simulink model "psbfilter"  (Simulink 6.0)
settings: Solver=ode45  SolverMode=SingleTasking  StartTime=0.0  StopTime=0.1  RelTol=1e-3  AbsTol=1e-6
libraries: powerlib2 x14
settings Model: Creator=patrice  LastModifiedBy=batserve  ExtModeTrigMode=oneshot  ExtModeArmWhenConnect=off  ExtModeAutoUpdateStatusClock=off
settings DataIOCC: LimitDataPoints=off  SignalLoggingName=sigsOut
settings OptimizationCC: BlockReduction=off  BooleanDataType=off
settings DebuggingCC: CheckExecutionContextPreStartOutputMsg=on  CheckExecutionContextRuntimeOutputMsg=on  SolverPrmCheckMsg=none
settings HardwareCC: TargetUnknown=on
settings RTWCC: TemplateMakefile=grt_unix.tmf

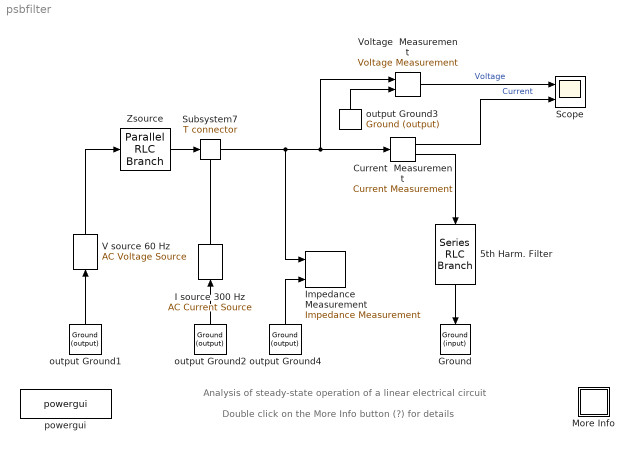
== system psbfilter ==
  note: Analysis of steady-state operation of a linear electrical circuit
  note: Double click on the More Info button (?) for details
  5th Harm. Filter : powerlib2/Elements/Series RLC Branch  Tag=PoWeRsYsTeMbLoCk  Orientation=down  a=1.27  b=107.42e-03  c=2.62e-06  mesure=None  PSBOutputType=1
  Current  Measurement : powerlib2/Measurements/Current Measurement  Tag=PoWeRsYsTeMmEaSuReMeNt  PhasorSimulation=off  OutputType=Magnitude  PSBOutputType=01  PSBequivalent=0
  Ground : powerlib2/Connectors/Ground (input)  Tag=PoWeRsYsTeMbLoCk  Orientation=down
  I source 300 Hz : powerlib2/Electrical Sources/AC Current Source  Tag=PoWeRsYsTeMbLoCk  Orientation=up  A=10  P=-30  F=300  stime=0  mesure=None  PSBOutputType=1
  Impedance  Measurement : powerlib2/Measurements/Impedance Measurement  Tag=PoWeRsYsTeMbLoCk  kz=1
  More Info : Subsystem
      mask Display: disp('?')
  Scope : Scope  NumInputPorts=2
      settings: TimeRange=0.1  YMin=-200~-10  YMax=200~10  DataFormat=Array
  Subsystem7 : powerlib2/Connectors/T connector  Tag=PoWeRsYsTeMbLoCk  PSBOutputType=1
  V source 60 Hz : powerlib2/Electrical Sources/AC Voltage Source  Tag=PoWeRsYsTeMbLoCk  Orientation=up  A=100  P=0  F=60  stime=0  mesure=None  PSBOutputType=1
  Voltage  Measurement : powerlib2/Measurements/Voltage Measurement  Tag=PoWeRsYsTeMmEaSuReMeNt  PhasorSimulation=off  OutputType=Magnitude  PSBOutputType=0  PSBequivalent=0
  Zsource : powerlib2/Elements/Parallel RLC Branch  Tag=PoWeRsYsTeMbLoCk  Description={'sdasdsad';'dsadsa'}  a=37.7  b=10e-03  c=0  mesure=None  PSBOutputType=1
  output Ground{1..4} (4 alike) : powerlib2/Connectors/Ground (output)  Tag=PoWeRsYsTeMbLoCk  Orientation=up  PSBOutputType=1
  powergui : powerlib2/powergui  Frange=0:2:1000  Ylog=off  Xlog=off  save=off  variable=ZData  ZoomFFT=on  StartTime=0.0  cycles=1  DisplayStyle=off  fundamental=60  FreqAxis=off  MaxFrequency=1000  frequencyindice=1  frequencyindicesteady=1  RmsSteady=1  display=off  Ts=0  methode=off  frequency=60  echomessages=off
  wires:
  V source 60 Hz/1 -> Zsource/1
  Zsource/1 -> Subsystem7/1
  I source 300 Hz/1 -> Subsystem7/Enable
  output Ground1/1 -> V source 60 Hz/1
  output Ground2/1 -> I source 300 Hz/1
  output Ground3/1 -> Voltage  Measurement/2
  5th Harm. Filter/1 -> Ground/1
  Current  Measurement/2 -> 5th Harm. Filter/1
  Voltage  Measurement/1 -> Scope/1  "Voltage"
  Subsystem7/1 -> Current  Measurement/1, Voltage  Measurement/1, Impedance  Measurement/1
  output Ground4/1 -> Impedance  Measurement/2
  Current  Measurement/1 -> Scope/2  "Current"

== system psbfilter/More Info ==
  note: 3
  note: 1
  note: Circuit Description
  note: Demonstration
  note: 2
  note: This demonstration illustrates use of the Powergui
      | and Impedance Measurement blocks to analyze the
      | steady-state operation of a linear electrical circuit
  note: Use the Powergui block to find the steady-sate  60Hz  and 300 Hz  components of  voltage and
      | current phasors.  The values of the 3 states (phasors and initial values)  can be also obtained
      | from the powergui block.
      |
      | Open the  scope and start the simulation from the Simulation/Start menu.
      | Notice that the simulation starts in steady-state.
      |
      | Using the Powergui block,  select Impedance vs Frequency Measurement. A new window opens.
      |
      | The measurement will be performed for the specified frequency range vector [ 0: 2:1000]  (0 to 1000 Hz
      | by steps of 2 Hz). Click on the Display button. The impedance is dispayed in a graphic window.
      | Notice the series resonance at 300 Hz corresponding to the tuned frequency of the  filter.
  note: A 5th harmonic filter is connected at a bus bar fed by a  60 Hz, 100 V inductive source.
      | A 5th harmonic (300 Hz, 1 A) current is injected at the bus bar.
      |
      | This linear system consists of 3 states (2 inductor currents and 1 capacitor voltage),
      |  2 inputs (Vs, Is) and 2 outputs (Current and Voltage Measurement).
      |
      | An Impedance Measurement  block is used to compute the impedance versus frequency of the circuit.
  note: G. Sybille (Hydro-Quebec)
